simulink model "dc_motor_position"  (R2020b)
settings: Solver=VariableStepAuto  StartTime=0.0  StopTime=0.2  RelTol=1e-3
values from neighbouring files (symbols this model uses):
  b = 3.5077E-6    [initial_values.sldd]
  J = 3.2284E-6    [initial_values.sldd]
  K = 0.0274    [initial_values.sldd]
  L = 2.75E-6    [initial_values.sldd]
  R = 4.0    [initial_values.sldd]
settings Model: Creator=Vrunda M Balgi  LastModifiedBy=Vrunda M Balgi

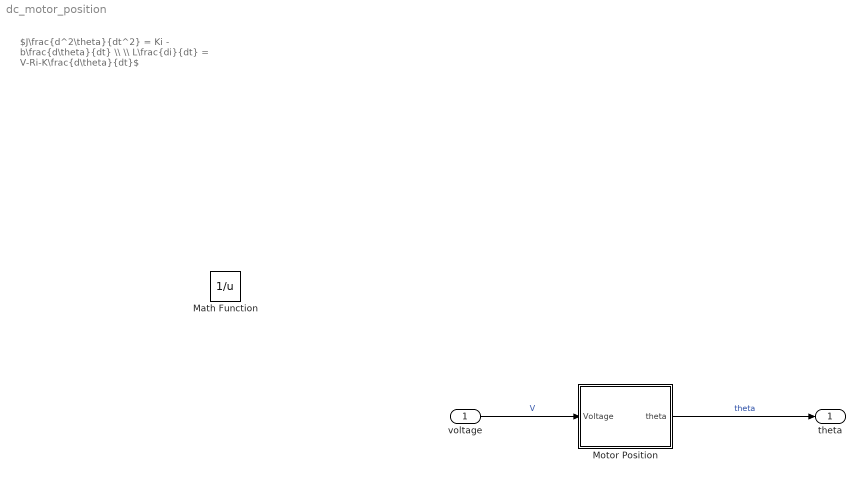
== system dc_motor_position ==
  note: $J\frac{d^2\theta}{dt^2} = Ki - b\frac{d\theta}{dt} \\ \\ L\frac{di}{dt} = V-Ri-K\frac{d\theta}{dt}$
  voltage : Inport
  Math Function : Math  Operator=reciprocal  SaturateOnIntegerOverflow=on
  Motor Position : Subsystem
  theta : Outport
  wires:
  voltage/1 -> Motor Position/1(Voltage)  "V"
  Motor Position/1(theta) -> theta/1  "theta"

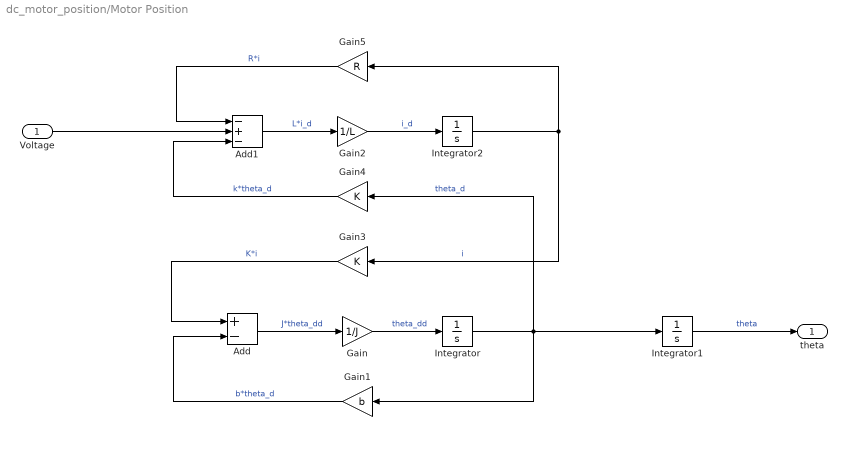
== system dc_motor_position/Motor Position ==
  Voltage : Inport
  Add : Sum  Inputs=+-
  Add1 : Sum  Inputs=-+-
  Gain : Gain  Gain=1/J
  Gain1 : Gain  Gain=b
  Gain2 : Gain  Gain=1/L
  Gain3 : Gain  Gain=K
  Gain4 : Gain  Gain=K
  Gain5 : Gain  Gain=R
  Integrator : Integrator
  Integrator1 : Integrator
  Integrator2 : Integrator
  theta : Outport
  wires:
  Gain5/1 -> Add1/1  "R*i"
  Gain2/1 -> Integrator2/1  "i_d"
  Gain3/1 -> Add/1  "K*i"
  Integrator/1 -> Gain1/1, Integrator1/1, Gain4/1  "theta_d"
  Gain4/1 -> Add1/3  "k*theta_d"
  Add/1 -> Gain/1  "J*theta_dd"
  Integrator2/1 -> Gain3/1, Gain5/1  "i"
  Gain1/1 -> Add/2  "b*theta_d"
  Gain/1 -> Integrator/1  "theta_dd"
  Integrator1/1 -> theta/1  "theta"
  Add1/1 -> Gain2/1  "L*i_d"
  Voltage/1 -> Add1/2
